simulink model "MCLV_V2_33EP256MC506_LongHurstMotor_sensored_V2"  (R2019a)
settings: Solver=FixedStepDiscrete  StartTime=0.0  StopTime=inf  FixedStep=.01  RelTol=1e-3  EnableMultiTasking=on
undefined symbols (not defined in the file or in its folder): A4, A8, B15, B9, C5, C6, D5, D8, F1, Max, MaxPer, ms, P20, P24, P41, P47, P53, P54, P97, Pin, PWMmax, Resol, us
libraries: MCHP_Blockset x20, simulink x4
(part 1 of 2)
settings Model: SimulationMode=external  ExtModeBatchMode=on  ExtModeTrigDuration=1  Creator=M91449  LastModifiedBy=Lubin Kerhuel
settings DataIOCC: LimitDataPoints=on  ReturnWorkspaceOutputs=off
settings OptimizationCC: DefaultParameterBehavior=Inlined  InlineInvariantSignals=on  LifeSpan=1
settings DebuggingCC: SFUnexpectedBacktrackingDiag=warning  SFNoUnconditionalDefaultTransitionDiag=warning  SFExecutionAtInitializationDiag=none  ArithmeticOperatorsInVariantConditions=warning
settings HardwareCC: ProdBitPerInt=16  ProdBitPerPointer=16  ProdBitPerSizeT=16  ProdBitPerPtrDiffT=16  ProdLargestAtomicInteger=Integer  ProdLargestAtomicFloat=None  ProdWordSize=16  ProdHWDeviceType=Generic->Custom
settings ModelReferenceCC: ModelReferenceNumInstancesAllowed=Single  PropagateSignalLabelsOutOfModel=off
settings SFSimCC: SimUseLocalCustomCode=off  MATLABDynamicMemAlloc=off
settings RTWCC: SystemTargetFile=MCHP_dsPIC_stf.tlc  TemplateMakefile=MCHP_dsPIC.tmf  Description=Microchip Embedded Target PIC24 dsPIC30 dsPIC33 (real-time)  GenerateReport=on  RTWUseLocalCustomCode=off  IncludeHyperlinkInReport=on  LaunchReport=on  GenerateTraceInfo=on  GenerateTraceReport=on  GenerateTraceReportSl=on  GenerateTraceReportSf=on  GenerateTraceReportEml=on  GenerateWebview=on  GenerateCodeMetricsReport=on  GenerateCodeReplacementReport=on
settings CodeAppCC: IgnoreCustomStorageClasses=off  MaxIdLength=255  StateflowObjectComments=on
settings STFCustomTargetCC: TargetLibSuffix=_lib.a  CodeReplacementLibrary=Microchip Code Replacement Library for dsPIC  IncludeMdlTerminateFcn=off  CombineOutputUpdateFcns=on  ERTCustomFileBanners=on  SupportContinuousTime=off  RemoveResetFunc=on  MATLABClassNameForMDSCustomization=Simulink.SoftwareTarget.ERTCustomization  GRTInterface=off  SystemTargetFile=MCHP_dsPIC_stf.tlc
settings ERTTargetCC: TargetLibSuffix=_lib.a  CodeReplacementLibrary=Microchip Code Replacement Library for dsPIC  MultiwordLength=2048  ParMdlRefBuildCompliant=off  CompOptLevelCompliant=off  ConcurrentExecutionCompliant=off  IncludeMdlTerminateFcn=off  SupportNonInlinedSFcns=on  ModelStepFunctionPrototypeControlCompliant=off  CPPClassGenCompliant=off  UseToolchainInfoCompliant=off  ExtMode=on  ExtModeStaticAlloc=on  ExtModeStaticAllocSize=512  ExtModeMexFile=ext_serial_win32_comm_no_acks  ExtModeMexArgs=1 4 115200  InlinedParameterPlacement=NonHierarchical  ERTSrcFileBannerTemplate=MCHP_dsPIC_code_template.cgt  ERTHdrFileBannerTemplate=MCHP_dsPIC_code_template.cgt  ERTDataSrcFileTemplate=MCHP_dsPIC_code_template.cgt  ERTDataHdrFileTemplate=MCHP_dsPIC_code_template.cgt  ERTCustomFileTemplate=MCHP_main.tlc  ConvertIfToSwitch=off  SuppressUnreachableDefaultCases=off
settings ConfigComp: CovMetricSettings=dw  CovHtmlReporting=on  CovSaveCumulativeToWorkspaceVar=on  CovSaveSingleToWorkspaceVar=on  CovExternalEMLEnable=off

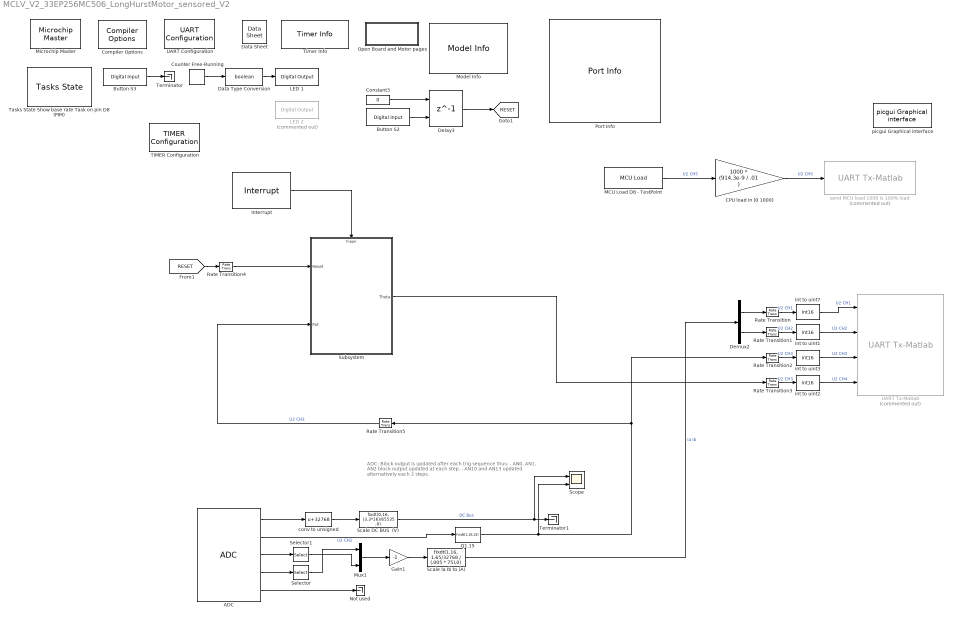
== system MCLV_V2_33EP256MC506_LongHurstMotor_sensored_V2 ==
  note: ADC:
      | Block output is updated after each trig sequence thus:
      | - AN0, AN1, AN2 block output updated at each step.
      | - AN10 and AN13 updated alternatively each 2 steps.
  ADC : MCHP_Blockset/Analog IO/ADC  Priority=5  ADC_REF=1  Mode=10 bits (allows exact simultaneous sampling)  FORM="sddd dddd dddd 0000  ==> Signed fractional"  ADC_R="< 5    kOhm"  nSAMPLECHANNELS=CH0 : CH1 : CH2 : CH3  nSAMPLECHANNELS_12bits=CH0 only  SIMULTANEOUS=Simultaneously on all Channels  ADxCSS=[10 13]  MUXA_CH0N=off  MUXA_CH123=Dynamic Options  MUXA_CH123_TXT=AN0 : AN1 : AN2  MUXB_CH0=AN1  MUXB_CH0N=on  MUXB_CH123=Dynamic Options  MUXB_CH123_TXT=AN0 : AN1 : AN2  SequenceRepeat=1  SequenceTiming=are done as fast as possible ; triggered by user define source  SSRC_SSRCG=Dynamic Options  SSRC_SSRCG_TXT=6  Update_BlockOutput=After all trig and conversion sequence  Trig_TimeStep=not synchronised with ADC [timer based...]  ADC_DMA_CHANNEL=Use Interrupt instead of DMA  SampleTime=0.01  Info=Total Time for Sample & Conversion : 8.9143e-06s including 3.4286e-07s (x 2) sample time.  MCHP_PORT={Analog Input 0}{AN0}15:2:A0;{Analog Input 1}{AN1}15:2:A1;{Analog Input 2}{AN2}15:2:B0;{Analog Input 10}{AN10}15:2:A12;{Analog Input 13}{AN13}15:2:E13;  MCHP_MASTERLINK=MCLV_V2_33EP256MC506_LongHurstMotor_sensored_V2/Microchip Master  ADC_TIMING=[8.9142857142857143663e-06]
      settings: SourceProductName=MPLAB Device Blocks for Simulink
  Button S2 : MCHP_Blockset/Digital IO/Digital Input  PORT=Dynamic Options  PORT_TXT="G   [ 6 : 9 ]"  PIN=7  PACK=off  SIMULTANEOUS=off  ORDERING=None  SampleTime=-1  MCHP_PORT={Digital In}{DIN}2:0:G7;  MCHP_MASTERLINK=MCLV_V2_33EP256MC506_LongHurstMotor_sensored_V2/Microchip Master
      settings: SourceProductName=MPLAB Device Blocks for Simulink
  Button S3 : MCHP_Blockset/Digital IO/Digital Input  PORT=Dynamic Options  PORT_TXT="G   [ 6 : 9 ]"  PIN=6  PACK=off  SIMULTANEOUS=off  ORDERING=None  SampleTime=.1  MCHP_PORT={Digital In}{DIN}2:0:G6;  MCHP_MASTERLINK=MCLV_V2_33EP256MC506_LongHurstMotor_sensored_V2/Microchip Master
      settings: SourceProductName=MPLAB Device Blocks for Simulink
  CPU load in [0 1000] : Gain  Gain=1000 * (914.3e-9 / .01 )  OutDataTypeStr=uint16
  Compiler Options : MCHP_Blockset/System Configuration/Compiler Options  Priority=1  LATEST_CMPLR=on  COMP_LIST=Dynamic Options  COMP_LIST_TXT=xc16 - v1.36  USE_64BIT_DOUBLE=off  MCHP_MULTITHREAD_COMPILATION=on  UseCustom_LinkerScript=off  MCHP_MASTERLINK=MCLV_V2_33EP256MC506_LongHurstMotor_sensored_V2/Microchip Master  OPTIMIZATION_LEVEL=3  OPTIMIZATION_FLTO=on  OPTIMIZATION_REORDER=off  UNROLL_LOOPS=on  PROCEDURAL_ABSTRACTION=off  MPLAB_LINKLIB=default  MPLAB_LINKLIB1=default  MCODE=is less than 32768 (faster)  MCONST=in data memory  MDATA=Use only memory below address 8192 (faster)  MSCALAR=Use only memory below address 8192 (faster)  MLARGEARRAY=off  MAGGREGATE=off  HEAP_SIZE=0  OMF=elf  DEBUG_INFO=off  ProduceHexOutput=on  AssemblyListing=off  NO_EDS_WARN=on  PRINT_STATISTICS=off
      settings: SourceProductName=MPLAB Device Blocks for Simulink
  Constant3 : Constant  Value=0  OutDataTypeStr=uint16  SampleTime=-1
  Counter Free-Running : simulink/Sources/Counter Free-Running  NumBits=1  tsamp=.1
  Data Sheet : MCHP_Blockset/System Info/Data Sheet  DOC_Type=datasheet  DOC_MCHP_Id=33EP256MC506_datasheet  DOC_FilePath=C:\Users\M91449\AppData\Local\Temp\70000657H.pdf  DOC_FileLastCheckTime="[2016              1             28             13             25         44.133]"  cpy_MCHP_Id=33EP256MC506  MCHP_MASTERLINK=MCLV_V2_33EP256MC506_LongHurstMotor_sensored_V2/Microchip Master
      settings: AttributesFormatString=%<cpy_MCHP_Id>  SourceProductName=MPLAB Device Blocks for Simulink
  Data Type Conversion : DataTypeConversion  OutDataTypeStr=boolean
  Delay3 : Delay  DelayLength=1  InitialCondition=1  ExternalReset=Falling  SampleTime=.1
      settings: InputPortMap=u0,r5
  Demux2 : Demux  Outputs=2
  Gain1 : Gain  Gain=-1  SaturateOnIntegerOverflow=on  OutDataTypeStr=Inherit: Same as input
  Interrupt : MCHP_Blockset/System Functions/Interrupt  Interruption=Dynamic Options  Interruption_TXT=TimerA  InterruptionLongDesc=TimerA  IntPriority=5  IntPriority_Info=5  StartupExecute=on  Status=OK  MCHP_MASTERLINK=MCLV_V2_33EP256MC506_LongHurstMotor_sensored_V2/Microchip Master  FPUNoSave=on  Triggered_Sub_TimeSource=is derived from model base rate  TrigsPeriod=0  TIMER_Resolution=Dynamic Options  TIMER_Resolution_TXT="Resol: 0.01429(us)  -  MaxPer: 0.936(ms)"  Info=0  SS_ASYNCHRONOUS_INTERRUPT=0  SS_TIMESOURCE=1  SS_AsyncTimerRes=-1  SS_AsyncTaskPriority=5  SS_ARCH=16
      settings: SourceProductName=MPLAB Device Blocks for Simulink
  LED 1 : MCHP_Blockset/Digital IO/Digital Output  PORT=Dynamic Options  PORT_TXT="D   [ 5  6  8 ]"  PIN=6  PACK=off  SIMULTANEOUS=off  READPREVIOUS=off  ORDERING=None  SampleTime=-1  MCHP_MASTERLINK=MCLV_V2_33EP256MC506_LongHurstMotor_sensored_V2/Microchip Master
      settings: SourceProductName=MPLAB Device Blocks for Simulink
  LED 2 : MCHP_Blockset/Digital IO/Digital Output  Commented=on  PORT=Dynamic Options  PORT_TXT="D   [ 5  6  8 ]"  PIN=5  PACK=off  SIMULTANEOUS=off  READPREVIOUS=off  ORDERING=None  SampleTime=-1  MCHP_MASTERLINK=MCLV_V2_33EP256MC506_LongHurstMotor_sensored_V2/Microchip Master
      settings: SourceProductName=MPLAB Device Blocks for Simulink
  MCU Load D8 - TestPoint : MCHP_Blockset/Profiling/MCU Load  MCULoadPin=Dynamic Options  MCULoadPin_TXT=D5 / Pin[53]  MCULoadMeasure=on  TIMER_Resolution=Dynamic Options  TIMER_Resolution_TXT="Resol: 0.9143(us)  -  Max: 59.9(ms)"  MCHP_PORT={MCU Load Pin}{MCU_Load}0:1:D5;  MCHP_TIMER_REQUEST={MCU_Load}{MCU_Load}21:5:0:0:[]:4194304;  MCHP_TIMER_RESULT=[3 65535 ]  MCHP_MASTERLINK=MCLV_V2_33EP256MC506_LongHurstMotor_sensored_V2/Microchip Master  MCHP_COMPILED_INFO="CompiledSampleTime= [0.010000000000000000208   0 ];CompiledInportDataTypes=[ ];CompiledInportDataWidth=[];"  Info="Timer 3:  Resol: 914.2857143(ns)  -  Max: 59.9186(ms)"  SampleTime=.01
      settings: SourceProductName=MPLAB Device Blocks for Simulink
  Microchip Master : MCHP_Blockset/System Configuration/Microchip Master  Priority=1  PICREF=33EP256MC506  TIMESTEP_REF="Timer  ( 0.01s + [-0.0045714%] ==> 0.0099995s )"  BUSYFLAG=Dynamic Options  BUSYFLAG_TXT=D8 / Pin[42]  PWRTEN=Not used  BOREN=Disable  BODENV=2.7V  BORV=Not used  FPWRT=128ms  DSBOREN=Enable ZPBOR during Deep Sleep Mode  DSLPBOR=Not used  MCLRE=Enabled  SMCLR=MCLR pin generates a normal system Reset  PMDL1WAY=Allow only one reconfiguration  RSTPRI=Device will obtain reset instruction from Primary flash  TEMP=Not used  SOSCSRC=Not used  SOSCSEL=Not used  IOL1WAY=Allow only one reconfiguration  ALTVREF=Not used  DISUVREG=Not used  DSSWEN=Not used  LPCFG=Not used  RTCBAT=Not used  VBTBOR=Not used  WUTSEL=Not used  POWERSAVE=off  FNOSC=Primary Oscillator (XT; HS; EC)  FPR=ECIO w/ PLL 16x  FOSFPR=HS3 w/PLL 16x  FOS=Primary Oscillator  FRANGE=High Range  OSCILLATOR_SELECT=Crystal / Ceramic resonator  OSCILLATOR_SELECT_spd=Crystal / Ceramic resonator  QUARTZ=8e6  QUARTZ_spd=8e6  POSCGAIN=2x gain setting  POSCBOOST=Boost the kick start of the oscillator  SOSCGAIN=2x gain setting  SOSCBOOST=Boost the kick start of the oscillator  ACTIV_PLL=on  ACTIV_PLL_spd=on  MIPS_DESIRED=70e6  MIPS_DESIRED_spd=70e6  FPLLMUL=Not used  FPLLIDIV=8x Divider  POSCFREQ=Not used  POSCMD=XT Crystal Oscillator Mode  POSCMOD=Primary Oscillator Disabled  MIPS=70 * 1e6  ACLKCON=Optimized for PWM resolution & ADC conversion speed  FPLLODIV=32x Divider  PLLKEN=Clock switch to PLL source will wait until the PLL lock signal is valid.  FCKSM=Both Clock switching and Fail-safe Clock Monitor are enabled  FCKSMEN=Sw Disabled; Mon Disabled  IESO=Start up with FRC; then switch  DSWDTPS=1:2^36  FWDTEN=Disable  FWDTWINSZ=Window size is 25%  FWPSA=1:512  FWPSA0=1:128  FWPSB=1:16  WDT=Disable  WDTPOST=1:32768  WDTPRE=1:128  WDTPS=1:32768  WINDIS=Watchdog Timer in Non-Window mode  WWDTEN=Non-Window mode  DSWDTEN=Enable DSWDT during Deep Sleep Mode  DSWDTOSC=Select LPRC as DSWDT Reference clock  FPBDIV=Not used  FSOSCEN=Enable SOSC  LPRCSEL=Not used  OSCIOFCN=Not used  OSCIOFNC=general purpose digital I/O pin  LVRCFG=Not used  PLL_96MHZ=Not used  PLL96MHZ=Not used  PLLDIV=Not used  WDTCLK=Not used  WDTCMX=Not used  WDTWIN=WDT Window is 25% of WDT period  XTCFG=24-32 MHz crystals  XTBST=Boost the kick-start  APL=Aux Flash Code protect is disabled  APLK=Aux Flash Write Protection or Code Protection is Enabled  AWRP=Auxiliary program memory is not write-protected  BSS=No Boot program Flash segment  BWP=Not used  BWRP=Boot Segment may be written  CP=Protection Disabled  EBS=No Boot EEPROM  ESS=No Segment Data EEPROM  GCP=General Segment Code protect is Disabled  GSS=General Segment Code protect is Disabled  GSS0=Not used  GSSK=General Segment Write Protection or Code Protection is Enabled  GWRP=General Segment may be written  PWP=Not used  RBS=No Boot RAM  RSS=No Secure RAM  SSS=No Secure Segment  SWRP=Secure segment may be written  WPCFG=Not used  WPDIS=Not used  WPEND=Not used  WPFP=Not used  ICESEL=Communicate on PGEC1/PGED1  ICS=Communicate on PGEC2 and PGED2  JTAGEN=Disable  COE=Not used  RES=Not used  DEBUG=Debugger is disabled  BACKBUG=Not used  BKBUG=Not used  ALTI2C=I2C mapped to SDA1/SCL1 pins  ALTI2C1=I2C1 mapped to SDA1/SCL1 pins  ALTI2C2=I2C2 mapped to SDA2/SCL2 pins  ALTI2C3=I2C3 mapped to SDA3/SCL3 pins  ALTQIO=QEA1; QEB1; INDX1 are selected as inputs to QEI1  ALTSS1=SS1A is selected as the I/O pin for SPI1  CMPPOL0=Hysteresis is applied to falling edge  CMPPOL1=Hysteresis is applied to falling edge  FCANIO=Not used  FETHIO=Default Ethernet I/O  FMIIEN=MII Enabled  FSRSSEL=Not used  FUSBIDIO=Controlled by the USB Module  FVBUSONIO=Not used  HPOL=PWM module high side output pins have active-high output polarity  HYST0=45 mV Hysteresis  HYST1=45 mV Hysteresis  I2C1SEL=Not used  LPOL=PWM module low side output pins have active-high output polarity  PWMPIN=PWM module pins controlled by PORT register at device Reset  RTCOSC=Not used  UPLLEN=USB PLL Disabled  UPLLIDIV=Not used  ATMOD8=Not used  ALTPMP=Not used  I2C2SEL=Not used  ALTADREF=Not used  ALTCVREF=Not used  PWMLOCK=PWM registers may be written without key sequence  INT_PRIORITY_DMA=0  MCHP_TIMER_REQUEST={Time Step}{TS}0:2:3:1:[]:700000;  MCHP_TIMER_RESULT=[1 10936.499999999987267 ]  MCHP_PORT={Busy Flag}{Busy}0:1:D8;  MCHP_PLLRegisters="[5    243  16385     -1     -1]"  MCHPVAR=MCHP.fcy.MIPS=70000000;MCHP.fcy.SYSCLK=70000000;MCHP.fcy.ADC=70000000;MCHP.fcy.Comparator=70000000;MCHP.fcy.I2C=70000000;MCHP.fcy.SPI=70000000;MCHP.fcy.UART=70000000;MCHP.fcy.Timers=70000000;MCHP.fcy.OC=70000000;MCHP.fcy.IC=70000000;MCHP.fcy.Ports=70000000;MCHP.fcy.QEI=70000000;MCHP.PowerSave=0;MCHP.TimeStepFactor=MCHP_Fun.Hex2num('3FEFFFA0215469B2');MCHP.TimeStep_Timer=1;MCHP.NTIMERS=5;MCHP.id.name='33EP256MC506';MCHP.id.N=reshape([33 256 506],1,3);MCHP.id.L=reshape({ 'EP','MC',''},1,3);MCHP.id.Arch=3;MCHP.periph.PPS.reg_RPINRx=reshape([-1 1 1 -1 -1 -1 1 -1 -1 -1 -1 -1 -1 -1 1 1 1 1 -1 -1 -1 -1 -1 -1 1 1 -1 -1 1 1 1 1 -1 -1 -1 -1 1 -1 1 -1 -1 -1 -1 -1 1 1 1 -1 -1 -1 -1 -1 1 -1 -1 -1 -1 -1 -1 -1 -1 -1 -1 -1 -1 -1 -1 -1 -1 -1 -1 -1 -1 -1 -1 1 -1 1 1 1],1,80);MCHP.PPS.dsPIC.RP=reshape([-1 -1 -1 -1 -1 -1 -1 -1 -1 -1 -1 -1 -1 -1 -1 -1 -1 -1 -1 -1 4 -1 -1 -1 -1 -1 -1 -1 -1 -1 -1 -1 -1 -1 -1 19 20 21 22 23 24 25 26 27 -1 -1 -1 -1 -1 -1 -1 -1 -1 -1 38 39 40 41 -1 -1 -1 -1 -1 -1 -1 -1 -1 -1 -1 -1 -1 -1 -1 -1 -1 -1 -1 -1 -1 -1 -1 -1 -1 -1 -1 -1 -1 -1 -1 -1 -1 -1 -1 -1 -1 -1 -1 81 -1 -1 -1 -1 -1 -1 -1 -1 -1 -1 -1 -1 -1 -1 -1 -1 -1 -1 -1 -1 102 -1 104],1,121);MCHP.PPS.dsPIC.RPI=reshape([-1 -1 -1 -1 -1 -1 -1 -1 -1 -1 -1 -1 -1 -1 -1 -1 -1 -1 -1 -1 -1 -1 -1 -1 8 9 -1 11 12 -1 -1 -1 16 17 18 -1 -1 -1 -1 -1 -1 -1 -1 -1 28 29 30 31 -1 -1 -1 35 36 37 -1 -1 -1 -1 42 -1 -1 -1 -1 -1 -1 -1 -1 -1 -1 -1 -1 -1 -1 -1 -1 -1 -1 -1 -1 -1 -1 -1 -1 -1 -1 -1 -1 -1 -1 -1 -1 -1 -1 -1 78 79 80 -1 -1 -1 -1 -1 -1 -1 -1 -1 -1 -1 -1 -1 -1 -1 -1 -1 -1 -1 -1 -1 -1 103 -1 105],1,122);MCHP.PPS.dsPIC.RPINR_list=reshape({ '1','INT1','INT2','INT3','INT4','T1CK','T2CK','T3CK','T4CK','T5CK','T6CK','T7CK','T8CK','T9CK','IC1','IC2','IC3','IC4','IC5','IC6','IC7','IC8','OCFA','OCFB','FLT1','FLT2','FLT3','FLT4','QEIA1','QEIB1','QEINDX1','QEIHOM1','QEIA2','QEIB2','QEINDX2','QEIHOM2','U1RX','U1CTS','U2RX','U2CTS','SDI1','SCK1_in','SS1_in','44','SDI2','SCK2_in','SS2_in','48','CSDIR','CSCK','COFS','52','C1RX','C2RX','U3RX','U3CTS','U4RX','U4CTS','SDI3','SCK3_in','SS3_in','62','SDI4','SCK4_in','SS4_in','66','IC9','IC10','IC11','IC12','IC13','IC14','IC15','IC16','OCFC','SYNCI1','SYNCI2','DTCMP1','DTCMP2','DTCMP3','DTCMP4','DTCMP5','DTCMP6','DTCMP7','FLT5','FLT6','FLT7','FLT8','89','SENT1','SENT2','92'},1,92);MCHP.PPS.dsPIC.RPOR_list=reshape({ '1','U1TX','U1RTS','U2TX','U2RTS','SDO1','SCK1_out','SS1_out','SDO2','SCK2_out','SS2_out','CSDO','CSCK','COFS','C1TX','C2TX','OC1','OC2','OC3','OC4','OC5','OC6','OC7','OC8','C1OUT','C2OUT','C3OUT','U3TX','U3RTS','U4TX','U4RTS','SDO3','SCK3_out','SS3_out','SDO4','SCK4_out','SS4_out','OC9','OC10','OC11','OC12','OC13','OC14','OC15','OC16','SYNCO1','SYNCO2','QEI1CCMP','QEI2CCMP','REFCLK','C4OUT','C5OUT','52','53','54','55','56','SENT1','SENT2'},1,59);MCHP.PPS.map_RPnR_RPORx=reshape([20 35 36 37 38 39 40 41 42 43 54 55 56 57 -1 97 -1 118 120],1,19);MCHP.Rx=reshape([13 15 21 -1 -1 58 -1 -1 -1 -1 -1 14 16 22 -1 -1 59 -1 -1 -1 -1 -1 -1 17 23 -1 -1 -1 -1 -1 -1 -1 -1 -1 18 35 -1 -1 -1 -1 -1 -1 -1 -1 33 32 36 -1 -1 -1 -1 -1 -1 -1 -1 -1 43 37 53 -1 -1 -1 -1 -1 -1 -1 -1 44 50 54 -1 -1 4 -1 -1 -1 -1 1 46 51 -1 -1 -1 5 -1 -1 -1 -1 31 48 52 42 -1 -1 6 -1 -1 -1 -1 34 49 55 -1 -1 -1 8 -1 -1 -1 -1 64 60 45 -1 -1 -1 -1 -1 -1 -1 -1 12 61 24 -1 -1 -1 -1 -1 -1 -1 -1 11 62 39 -1 27 -1 -1 -1 -1 -1 -1 -1 63 47 -1 28 -1 -1 -1 -1 -1 -1 -1 2 -1 -1 29 -1 -1 -1 -1 -1 -1 -1 3 40 -1 30 -1 -1 -1 -1 -1 -1],11,16);MCHP.ADC.ANtype=reshape([3 0],1,2);MCHP.ADC.ADCONx=reshape([47103 59391 40959 263 0 0],1,6);MCHP.ADC.ADCHS_0=reshape([40863 1799],1,2);MCHP.ADC.Flags=reshape([1 0],1,2);MCHP.ADC.Buffer=reshape([16 -1],1,2);MCHP.ADC.port=reshape([0 1 16 17 18 19 32 33 34 11 12 43 76 77 78 79 -1 -1 -1 -1 -1 -1 -1 -1 -1 -1 -1 -1 -1 -1 -1 -1 -1 -1 -1 -1 -1 -1 -1 -1 -1 -1 -1 -1 -1 -1 -1 -1 -1 -1 -1 -1 -1 -1 -1 -1 -1],1,57);MCHP.ADC.port_ALT=reshape([-1 -1 -1 -1],1,4);MCHP.ADC.port_VrefP=17;MCHP.ADC.port_VrefM=16;MCHP.ADC.port_AVdd=-1;MCHP.ADC.port_AVss=-1;MCHP.ADC.ADCDATA=reshape([0 0 0 0 0 0 0 0 0 0 0 0 0 0 0 0 0 0 0 0 0 0 0 0 0 0 0 0 0 0 0 0 0 0 0 0 0 0 0 0 0 0 0 0 0 0 0 0 0 0 0 0 0 0 0 0 0],1,57);MCHP.ADC.HS_SAR.TRGSRC=reshape([0 0 0 0 0 0 0 0 0 0 0 0 0 0 0 0 0 0 0 0 0 0 0 0 0 0],1,26);MCHP.ADC.HS_SAR.nFilters=0;MCHP.ADC.HS_SAR.nDedicatedCore=0;MCHP.ADC.HS_SAR.CALIBRATION=0;MCHP.ADC.HS_SAR.ADCON1L=-1;MCHP.memory.RAM=32768;MCHP.memory.RAM_XBegin=4096;MCHP.memory.RAM_YBegin=20480;MCHP.memory.RAM_dma=reshape([-1 -1],1,2);MCHP.memory.FLASH_ECC=0;MCHP.DMA.Num=4;MCHP.DMA.CNTmax=16383;MCHP.QEI.QEICONx=reshape([49023 -1 -1 -1 -1 -1],1,6);MCHP.QEI.QEItype=1;MCHP.QEI.Port_QEI_INDX=reshape([-1 -1],1,2);MCHP.QEI.Port_QEI_QEA=reshape([-1 -1],1,2);MCHP.QEI.Port_QEI_QEB=reshape([-1 -1],1,2);MCHP.QEI.Port_QEI_UPDN=reshape([-1 -1],1,2);MCHP.INT.Port=reshape([23 32767 32767 -1 -1],1,5);MCHP.PWM_HS.Flags=reshape([3 1 0],1,3);MCHP.PWM.port_FLT=reshape([-1 -1 -1 34 43 -1 -1 -1 -1 -1 -1 -1 -1 -1 -1 -1 -1 -1 -1 -1 -1 -1 -1 -1 -1 -1 -1 -1 -1 -1 -1 -1 20],1,33);MCHP.PWM.PWMRef=-1;MCHP.PWM.Flag=0;MCHP.PWM.Port_PWM_l=reshape([31 -1 29 -1 27 -1 -1 -1 -1 -1 -1 -1 -1 -1 -1 -1 -1 -1 -1 -1 -1 -1 -1 -1],2,12);MCHP.PWM.Port_PWM_h=reshape([30 -1 28 -1 26 -1 -1 -1 -1 -1 -1 -1 -1 -1 -1 -1 -1 -1 -1 -1 -1 -1 -1 -1],2,12);MCHP.PWM_HS_FEP.nEVTOUT=-1;MCHP.IC.Port=reshape([32767 32767 32767 32767 0 0 0 0 0 0 0 0 0 0 0 0],1,16);MCHP.IC.type=1;MCHP.OC.Port=reshape([32767 32767 32767 32767 0 0 0 0 0 0 0 0 0 0 0 0],1,16);MCHP.OC.type=1;MCHP.CN.Port=reshape([-1 -1 -1 -1 -1 -1 -1 -1 -1 -1 -1 -1 -1 -1 -1 -1 -1 -1 -1 -1 -1 -1 -1 -1 -1 -1 -1 -1 -1 -1 -1 -1 -1 -1 -1 -1 -1 -1 -1 -1 -1 -1 -1 -1 -1 -1 -1 -1 -1 -1 -1 -1 -1 -1 -1 -1 -1 -1 -1 -1 -1 -1 -1 -1 -1 -1 -1 -1 -1 -1 -1 -1 -1 -1 -1 -1 -1 -1 -1 -1 -1 -1 -1 -1 -1],1,85);MCHP.CN.PullUp=reshape([8083 65535 49151 352 61440 3 960 0 0 0 0],1,11);MCHP.CN.type=1;MCHP.CN.Flag_PullDown=1;MCHP.SPI.Refs=reshape([1 2 0 0 0 0],1,6);MCHP.SPI.SPIxCON1=8191;MCHP.SPI.SPIxCON2=57347;MCHP.SPI.Port_SDI=reshape([9 -1 -1 -1 -1 -1],1,6);MCHP.SPI.Port_SDO=reshape([4 -1 -1 -1 -1 -1],1,6);MCHP.SPI.Port_SCK=reshape([35 -1 -1 -1 -1 -1],1,6);MCHP.SPI.Port_SS=reshape([16 -1 -1 -1 -1 -1],1,6);MCHP.I2C.Refs=reshape([1 2 0 0 0],1,5);MCHP.I2C.I2CxCON=49151;MCHP.I2C.NewRegName=1;MCHP.I2C.Port_SDA=reshape([36 8 -1 -1 -1],1,5);MCHP.I2C.Port_SCL=reshape([37 20 -1 -1 -1],1,5);MCHP.I2C.Port_ASDA=reshape([25 21 -1 -1 -1],1,5);MCHP.I2C.Port_ASCL=reshape([24 22 -1 -1 -1],1,5);MCHP.I2C.Fuse_Port_SCL_SDA=reshape([3 1 4 1 -1 -1 -1 -1 -1 -1],2,5);MCHP.I2C.Fuse_Port_ASCL_ASDA=reshape([3 2 4 2 -1 -1 -1 -1 -1 -1],2,5);MCHP.SCCP.nSCCP=0;MCHP.SCCP.MCCP=reshape([0 0 0 0 0 0 0 0 0],1,9);MCHP.PGA.Port_PGA1P=reshape([-1 -1 -1 -1],1,4);MCHP.PGA.Port_PGA1N=reshape([-1 -1 -1 -1],1,4);MCHP.PGA.Port_PGA2P=reshape([-1 -1 -1 -1],1,4);MCHP.PGA.Port_PGA2N=reshape([-1 -1 -1 -1],1,4);MCHP.PGA.Num=2;MCHP.HS_AnalogComparator.Port_CMP1=reshape([-1 -1 -1 -1],1,4);MCHP.HS_AnalogComparator.Port_CMP2=reshape([-1 -1 -1 -1],1,4);MCHP.HS_AnalogComparator.Port_CMP3=reshape([-1 -1 -1 -1],1,4);MCHP.HS_AnalogComparator.Port_CMP4=reshape([-1 -1 -1 -1],1,4);MCHP.HS_AnalogComparator.PORT_EXTREFx=reshape([-1 -1],1,2);MCHP.HS_AnalogComparator.Port_DACOUTx=reshape([-1 -1],1,2);MCHP.HS_AnalogComparator.Num=2;MCHP.Comp.Port_CVrefin=-1;MCHP.Comp.Port_CVref=-1;MCHP.Comp.Port_CVref1O=24;MCHP.Comp.Port_CVref2O=4;MCHP.Comp.Port_CxOUT=reshape([32767 32767 32767 32767 -1],1,5);MCHP.Comp.Port_OAxOUT=reshape([17 0 32 -1 -1],1,5);MCHP.Comp.Port_CxINP=reshape([18 1 34 32 -1],1,5);MCHP.Comp.Port_CxINM=reshape([19 43 -1 -1 16 76 -1 -1 33 77 -1 -1 33 -1 -1 -1 -1 -1 -1 -1],4,5);MCHP.Comp.Port_OAxINP=reshape([-1 -1 -1 -1 -1],1,5);MCHP.Comp.Port_OAxINM=reshape([-1 -1 -1 -1 -1],1,5);MCHP.Comp.nComp=reshape([4 0 0],1,3);MCHP.Comp.OpAmp=7;MCHP.Comp.CVRCON=reshape([17663 0],1,2);MCHP.CDAC.Port_DACx=reshape([-1 -1 -1],1,3);MCHP.CDAC.nCDAC=0;MCHP.UART.port_Rx=reshape([32767 32767 -1 -1 -1 -1],1,6);MCHP.UART.port_Tx=reshape([32767 32767 -1 -1 -1 -1],1,6);MCHP.UART.port_ARx=reshape([-1 -1],1,2);MCHP.UART.port_ATx=reshape([-1 -1],1,2);MCHP.UART.port_RTS=reshape([34 76 -1 -1 -1 -1],1,6);MCHP.UART.port_CTS=reshape([43 77 -1 -1 -1 -1],1,6);MCHP.UART.reg_UxMODE=reshape([48127 48127 -1 -1 -1 -1],1,6);MCHP.UART.reg_UxSTA=reshape([61439 61439 -1 -1 -1 -1],1,6);MCHP.modsrc.DOS_02551_cpu_16bit_v7=0;MCHP.modsrc.DOS_01520_wdt_dmt_upb_v1_16bit=0;MCHP.modsrc.DOS_02359a_sent_j2716_upb_v1=0;MCHP.modsrc.DOS_02672_math_progcrc_upb_v1_16bit=0;MCHP.modsrc.DOS_01577_cla_clc_upb_v1=0;MCHP.modsrc.DOS_02915_ecc_v2=0;MCHP.modsrc.DOS_02673_tmr_classa_upb_v1_16bit=0;MCHP.modsrc.DOS_01494_qei_32b_upb_v1_16bit=0;MCHP.modsrc.DOS_02552_msi_upb_v1_Master=0;MCHP.modsrc.DOS_01441_i2c_upb_v1_16bit_TLAH=0;MCHP.modsrc.DOS_03076_uart_protocol_upb_v1_16bit=0;MCHP.modsrc.DOS_01482=0;MCHP.modsrc.DOS_01483_pwm_16bit=0;MCHP.modsrc.DOS_03247_CAN_FD_UPB_V2_16_bit=0;MCHP.modsrc.DOS_02497_WACV=0;MCHP.modsrc.DOS_02316_nvm_ctrl_v1_16bit=0;MCHP.modsrc.DOS_02653_afe_current_bias_ctrl_upb_v1_16bit=0;MCHP.modsrc.DOS_01459_ptg_pc_upb_v1_16bit=0;MCHP.modsrc.DOS_01512_ccp_mccp_upb_v1_16bit=0;MCHP.modsrc.DOS_02519_dma_sfr_16bit_v2=0;MCHP.modsrc.DOS_02508c11=0;MCHP.modsrc.DOS_02475_dac_pdm_nbit_upb_v1_16bit=0;MCHP.modsrc.DOS_02467_gpio_upb_v1_16bit=0;MCHP.modsrc.DOS_00805_rst_integration_v4=0;MCHP.modsrc.DOS_02659_clk_sib_v12=0;MCHP.modsrc.DOS_02674_wdt_upb_v1_16bit=0;MCHP.modsrc.DOS_01407=0;MCHP.modsrc.DOS_02552_msi_upb_v1_Slave=0;MCHP.modsrc.DOS_02593_amp_pga_ctrl_pb_v2_16bit=0;MCHP.modsrc.DOS_01461_afe_ctmu_con_upb_v1_16bit=0;MCHP.modsrc.DOS_02497_WACA=0;MCHP.modsrc.DOS_02478_uart_irda_upb_v1_16bit=0;MCHP.modsrc.DOS_00929=1;MCHP.modsrc.DOS_01198=1;MCHP.modsrc.DOS_03029_WACH=0;MCHP.modsrc.DOS_02472_ppi_pmp16_upb_v1_16bit=0;MCHP.modsrc.DOS_02949_WACG=0;MCHP.modsrc.DOS_03349_amp_pad_opamp_ctrl_upb_v1=0;MCHP.modsrc.DOS_02237_osc_dco_ctrl_upb_v1_16bit=0;MCHP.modsrc.DOS_03662_WACU=0;MCHP.modsrc.DOS_03994_WAC07_Module=0;MCHP.modsrc.DOS_00794=1;MCHP.modsrc.DOS_00931=1;MCHP.modsrc.DOS_00932=1;MCHP.modsrc.DOS_00942=1;MCHP.modsrc.DOS_00938=1;MCHP.modsrc.DOS_00996=1;MCHP.modsrc.DOS_00997=1;MCHP.modsrc.DOS_00998=1;MCHP.modsrc.DOS_00209=0;MCHP.modsrc.DOS_01555_adc=0;MCHP.modsrc.DOS_01293=1;MCHP.modsrc.DOS_00828=0;MCHP.modsrc.DOS_01116=1;MCHP.modsrc.DOS_01017_RPORx=1;MCHP.modsrc.DOS_01017_RPINRx=1;MCHP.modsrc.DOS_01555_nvm_tsmc18_v2_16bit=0;MCHP.modsrc.DOS_00804=1;MCHP.modsrc.DOS_00826=1;MCHP.modsrc.DOS_01555_TLAK_PMDx=0;MCHP.modsrc.DOS_01555_TLAK_INT_=0;MCHP.modsrc.DOS_00933=1;MCHP.modsrc.DOS_01555=0;MCHP.modsrc.DOS_01555_ptg=0;MCHP.modsrc.DOS_00958=1;MCHP.modsrc.DOS_01117_PORTx=1;MCHP.modsrc.DOS_00999=0;MCHP.modsrc.DOS_01041=1;MCHP.modsrc.DOS_00892=1;MCHP.modsrc.DOS_01287_TLAC_PMDx=1;MCHP.modsrc.DOS_01287_TLAC_INT_=1;MCHP.modsrc.DOS_01424=1;MCHP.modsrc.DOS_01332=1;MCHP.modsrc.DOS_01468_PMBA_current_source=0;MCHP.modsrc.DOS_02291_PGA=0;MCHP.modsrc.DOS_01467_Comparator=0;MCHP.modsrc.DOS_01498_TLAY=0;MCHP.modsrc.DOS_00993_PLL_120MHz=0;MCHP.modsrc.DOS_01332_ptg_pc_v1=0;MCHP.modsrc.DOS_00958_pwm_TLAY=0;MCHP.modsrc.TLAY_IOPorts=0;MCHP.modsrc.DOS_00929q=0;MCHP.modsrc.DOS_02415_spi_v5=0;MCHP.modsrc.DOS_RPINRx_16bit_2=0;MCHP.modsrc.DOS_01497_TLAH_PMDx=0;MCHP.modsrc.DOS_02550_TLAL_INT=0;MCHP.modsrc.DOS_00958_pwm_TLAH=0;MCHP.modsrc.DOS_01287_TLAH_INT_=0;MCHP.modsrc.DOS_01113=0;MCHP.modsrc.DOS_01017_PMDx=0;MCHP.modsrc.DOS_00927=0;MCHP.modsrc.DOS_01080=0;MCHP.modsrc.DOS_00794_cpu_16bit_v3=0;MCHP.modsrc.DOS_02192_TLCD_PMDx=0;MCHP.modsrc.DOS_02192_TLCD_INT_=0;MCHP.modsrc.DOS_02192_cmp=0;MCHP.modsrc.DOS_00958_pwm_TLCD=0;MCHP.modsrc.DOS_02192_PORTx_TLCD=0;MCHP.modsrc.DOS_00936=0;MCHP.modsrc.DOS_00995=0;MCHP.modsrc.DOS_00546=0;MCHP.modsrc.DOS_00474=0;MCHP.modsrc.DOS_02481_WACJ_MC_Config=0;MCHP.modsrc.DOS_02569_pfm_cache_ocp_v1=0;MCHP.modsrc.DOS_02819_pfm_ctrl_32bit_upb_v2=0;MCHP.modsrc.DOS_02674_wdt_upb_v1_32bit=0;MCHP.modsrc.DOS_01520_wdt_dmt_upb_v1=0;MCHP.modsrc.DOS_02869_icd_jtag_bvci_upb_v2=0;MCHP.modsrc.DOS_02823_WACJ_clk_cru_upb_v2=0;MCHP.modsrc.DOS_01423_RPINRx=0;MCHP.modsrc.DOS_02481_RPORx=0;MCHP.modsrc.DOS_02511_pwr_sib_upb_v1_32bit=0;MCHP.modsrc.DOS_02481_WACJ_MC_int_evic_v3=0;MCHP.modsrc.DOS_01500_dma_bvci_v2=0;MCHP.modsrc.DOS_02141_tmr_classa_pb_v2=0;MCHP.modsrc.DOS_02815_tmr_classb_upb_v1=0;MCHP.modsrc.DOS_00740_icap_pb_v1=0;MCHP.modsrc.DOS_00749_ocmp_pb_v1=0;MCHP.modsrc.DOS_01441_i2c_upb_v1_32bit=0;MCHP.modsrc.DOS_01329_spi_pb_v2=0;MCHP.modsrc.DOS_02478_uart_irda_upb_v1_32bit=0;MCHP.modsrc.DOS_02514_dfm_strl_sst_upb_v1=0;MCHP.modsrc.DOS_01477_pwm_mc_upb_v1=0;MCHP.modsrc.DOS_01459_ptg_pc_upb_v1_SIC=0;MCHP.modsrc.DOS_01494_qei_32b_upb_v1=0;MCHP.modsrc.DOS_01427_cmp_control_upb_v1_32bit=0;MCHP.modsrc.DOS_01445_dac_nbit__control_upb_v1_32bit=0;MCHP.modsrc.DOS_01461_afe_ctmu_con_upb_v1=0;MCHP.modsrc.DOS_02472_ppi_pmp16_upb_v1=0;MCHP.modsrc.DOS_02467_gpio_ports_upb_v1=0;MCHP.modsrc.DOS_01152_can_bvci_v1=0;MCHP.modsrc.DOS_02508_adc_sar_ctrl_upb_v1_PIC32MK=0;MCHP.modsrc.DOS_02813a_usb_otgcore_pb_v3=0;MCHP.modsrc.DOS_01261_tmr_rtcc_pb_v2=0;MCHP.modsrc.DOS_01475_lpwr_deep_sleep_ctrl_v2=0;MCHP.modsrc.DOS_EIP_00136_ssx_v1=0;MCHP.modsrc.DOS_02481_WACK_MC_Config=0;MCHP.modsrc.DOS_03088_pfm_cache_ocp_v2_WACK=0;MCHP.modsrc.DOS_02823_WACN_clk_cru_upb_v2=0;MCHP.modsrc.DOS_02907_WACK_MC_int_evic_v3=0;MCHP.modsrc.DOS_03554_cmp_control_upb_v2_32bit=0;MCHP.modsrc.DOS_03247_can_fd_upb_v2_pic32mk=0;MCHP.modsrc.DOS_02787_WACD_Config=0;MCHP.modsrc.DOS_00800_dac_4bit_ctrl_pb_v1=0;MCHP.modsrc.DOS_01539_icd_jtag_pb_v2=0;MCHP.modsrc.DOS_02823_clk_cru_upb_v2=0;MCHP.modsrc.DOS_01423_RPORx=0;MCHP.modsrc.DOS_02907_WACD_int_evic_v3=0;MCHP.modsrc.DOS_00734_uart_irda_pb_v1=0;MCHP.modsrc.DOS_00687_tmr_classa_pb_v1=0;MCHP.modsrc.DOS_00745_tmr_classb_pb_v1=0;MCHP.modsrc.DOS_02508_adc_sar_ctrl_upb_v1=0;MCHP.modsrc.DOS_00866_cmp_control_pb_v2=0;MCHP.modsrc.DOS_01114_eth_bvci_v1=0;MCHP.modsrc.DOS_02831_usb_clk_rst_v2=0;MCHP.modsrc.DOS_01643_pfm_cache_ahb_v2=0;MCHP.modsrc.DOS_EIP_00206r5_sqi_v2=0;MCHP.modsrc.DOS_EIP_00124_usb_hs_otgcore_v1=0;MCHP.modsrc.DOS_EIP_00218_math_rng_ahbs_v2=0;MCHP.modsrc.DOS_EIP_00109_ebi_v1=0;MCHP.modsrc.DOS_EIP_00158_crypto_v1=0;MCHP.PortBase=16;MCHP.PortPrefixe='P';MCHP.clock.PBxDIV=-1;  MCHP_CRC=6863099  BTMODE=Not used  RES1=Not used  PLLSS=Not used  RES2=Not used  ALTCMPI=Not used  BOREN1=Not used  ALTRB6=Not used  RETCFG=Not used  DFMCY=Not used  BSS2=No Boot Segment  BSEN=No Boot Segment  CWRP=Configuration Segment may be written  CSS=No Protection (other than CWRP)  AIVTDIS=Disable Alternate Vector Table  BSLIM=Not used  WDTEN=Disable  BTSWP=BOOTSWP instruction is disabled  DBCC=No Cross Connection between DAC outputs  CTXT1=Not Assigned  CTXT2=Not Assigned  SEQNUM=Not used  nSEQNUM=Not used  BOREN0=Enabled  DMTIVT=Not used  DMTCNT=2^31 (2147483648)  DMTEN=Dead Man Timer is Disabled and can be enabled by software  ON=Not used  USERID=Not used  RESERVED1=Not used  PGL1WAY=Allow only one reconfiguration  FPLLRNG=34-68 MHz Input  FPLLICLK=FRC is input to the System PLL  FPLLMULT=PLL Multiply by 128  UPLLFSEL=USB PLL input is 24 MHz  DMTINTV=Window/Interval value is 127/128 counter value  WDTSPGM=WDT stops during Flash programming  FDMTEN=Deadman Timer is disabled  TRCEN=Trace features in the CPU are enabled  BOOTISA=Boot code and Exception code is MIPS32  FECCCON=ECC and Dynamic ECC are disabled (ECCCON bits are writable)  EXTDDRSIZE=Not used  FSLEEP=Flash is powered down when the device is in Sleep mode  DBGPER=Allow CPU access to all permission regions  EJTAGBEN=Normal EJTAG functionality  TSEQ=Not used  CSEQ=Not used
      settings: SourceProductName=MPLAB Device Blocks for Simulink
  Model Info : simulink/Model-Wide Utilities/Model Info  Frame=on  DisplayStringWithTags=|  HorizontalTextAlignment=Left  LeftAlignmentValue=0.02
      | Long hust motor with:
      | M1 - Black
      | M2 - Red
      | M3 - White
      | 
      | Encoder on HA - HB 
      | HA: Blue wire
      | HB: White wire
  Mux1 : Mux  Inputs=2
  Not used : Terminator
  Open Board and Motor pages : Subsystem
      settings: OpenFcn=|
      | web('www.microchip.com/DevelopmentTools/ProductDetails.aspx?PartNO=DM330021-2','-browser');
      | pause(1);
      | web('http://www.microchipdirect.com/productsearch.aspx?keywords=AC300020','-browser');
      | pause(1);
      | web('www.microchipdirect.com/ProductSearch.aspx?keywords=AC300022','-browser');
      mask Display: disp('Open tools\nWebpage');
  Port Info : MCHP_Blockset/System Info/Port Info  MCHP_MASTERLINK=MCLV_V2_33EP256MC506_LongHurstMotor_sensored_V2/Microchip Master
      settings: SourceProductName=MPLAB Device Blocks for Simulink
  Q1.15 : DataTypeConversion  OutDataTypeStr=fixdt(1,16,15)  ConvertRealWorld=Stored Integer (SI)
  Rate Transition : RateTransition
  Rate Transition1 : RateTransition
  Rate Transition2 : RateTransition
  Rate Transition3 : RateTransition  Deterministic=off
  Rate Transition4 : RateTransition  Deterministic=off
  Rate Transition5 : RateTransition  Deterministic=off
  Scale DC BUS  (V) : DataTypeConversion  OutDataTypeStr=fixdt(0,16, (3.3*16)/65535 ,0)  ConvertRealWorld=Stored Integer (SI)
  Scale Ia Ib to (A) : DataTypeConversion  OutDataTypeStr=fixdt(1,16, 1.65/32768 / (.005 * 75),0)  ConvertRealWorld=Stored Integer (SI)
  Scope : Scope  NumInputPorts=2
  Selector : Selector  InputPortWidth=2  IndexOptions=Index vector (dialog)  Indices=2  OutputSizes=1
  Selector1 : Selector  InputPortWidth=2  IndexOptions=Index vector (dialog)  Indices=2  OutputSizes=1
  Subsystem : Subsystem
  TIMER Configuration : MCHP_Blockset/Timers/TIMER Configuration  TIMER_Name=TimerA  TIMER_CustomName=pouet_p  TIMER_Ressource=Dynamic Options  TIMER_Ressource_TXT=No constraints [Prefered]  TIMER_Ressource_Custom=[1]  DoNotSetupChk=off  TIMER_PeriodChk=off  TIMER_Period=50e-6  TIMER_Resolution=Dynamic Options  TIMER_Resolution_TXT="Resol: 3.657(us)  -  MaxPer: 240(ms)"  TIMER_Interrupt=off  TIMER_Use=Read only  TIMER_ShareChk=on  MCHP_TIMER_REQUEST="{TimerA}{TmrCfg}20:2:3:0:[1  2  3  4  5]:3500;"  MCHP_TIMER_RESULT=[2 3498.9999999999990905 ]  MCHP_USER_INTERRUPTS={T2}{TimerA}{TimerA}{VectorName(T2Interrupt) Priority(-1) };  MCHP_MASTERLINK=MCLV_V2_33EP256MC506_LongHurstMotor_sensored_V2/Microchip Master  Info="Timer 2:  Resol: 14.28571429(ns)  -  Per: 50(us)  -  Max value: 936.214(us)"
      settings: SourceProductName=MPLAB Device Blocks for Simulink
  Tasks State Show base rate Task on pin D8 (PIM) : MCHP_Blockset/Profiling/Tasks State  TasksPin=D8  MCHP_PORT={Task D1 Running}{Task D1}15:1:D8;  MCHP_MASTERLINK=MCLV_V2_33EP256MC506_LongHurstMotor_sensored_V2/Microchip Master
      settings: SourceProductName=MPLAB Device Blocks for Simulink
  Terminator : Terminator
  Terminator1 : Terminator
  Timer Info : MCHP_Blockset/System Info/Timer Info  MCHP_MASTERLINK=MCLV_V2_33EP256MC506_LongHurstMotor_sensored_V2/Microchip Master
      settings: SourceProductName=MPLAB Device Blocks for Simulink
  UART Configuration : MCHP_Blockset/BUS UART/UART Configuration  UART_REF=2  BAUD_Choice=Dynamic Options  BAUD_Choice_TXT="115200         [-0.06%]"  BAUD_Choice_IR=Dynamic Options  BAUD_Choice_IR_TXT=[]  BAUD_Custom=115200  INT_PRIORITY=0  ALT_IO=on  PIN_RX=Dynamic Options  PIN_RX_TXT=C5 / P53 / Pin[37]  PIN_TX=Dynamic Options  PIN_TX_TXT=F1 / P97 / Pin[59]  MCHP_PORT="{UART2  Rx}{U2RX}3:0:P53;{UART2  Tx}{U2TX}3:1:P97;"  MCHP_MASTERLINK=MCLV_V2_33EP256MC506_LongHurstMotor_sensored_V2/Microchip Master  MCHP_COM_ExtPil=on  TX_IMPLEMENTATION=Circular Buffer  TX_IMPLEMENTATION_default=Circular Buffer  TX_INT_PRIORITY=5  TX_INT_WHEN=is empty & last char is sent  TX_INT_WHEN_default=is empty & last char is sent  TX_CIRCULAR_SIZE=256  TX_DMA_CHANNEL="0   (Lowest Priority)"  TX_DMA_SIZE=60  TX_TASK_PROTECTION=Delay tasks (default)  TX_INTERRUPT_PROTECTION=Do not send on conflict (default)  TX_INTERRUPT_PROTECTION_default=Do not send on conflict (default)  RX_IMPLEMENTATION=Circular Buffer  RX_IMPLEMENTATION_default=Circular Buffer  RX_INT_PRIORITY=5  RX_INT_WHEN=is 3/4 fulll (contains 3 data characters)  RX_CIRCULAR_SIZE=256  RX_DMA_CHANNEL=0  RX_DMA_SIZE=0  DuplexMode=Full duplex (default)  PIN_RX_Inv=off  PIN_TX_Inv=off  PIN_RXTX_Inv=off  ParityBit=No parity (default)  StopBit=1 stop bit (default)  IRDA=off  FlowControl=None  PIN_CTS=Dynamic Options  PIN_CTS_TXT=A4 / P20 / Pin[33]  PIN_RTS=Dynamic Options  PIN_RTS_TXT=A4 / P20 / Pin[33]  InitSequence_chkbox=off  BAUD_Choice_InitSeq=Dynamic Options  BAUD_Choice_InitSeq_TXT="110         [-0.00%]"  BAUD_Choice_IR_InitSeq=Dynamic Options  BAUD_Choice_IR_InitSeq_TXT=0  BAUD_Custom_InitSeq=0  InitSequence='Hello World'
      settings: SourceProductName=MPLAB Device Blocks for Simulink
  UART Tx-Matlab : MCHP_Blockset/BUS UART/UART Tx-Matlab  Commented=on  UART_REF=2  CHANNELS=[1 2 3 4 ]  AllOrNothing=on  SampleTime=.001  MCHP_MASTERLINK=MCLV_V2_33EP256MC506_LongHurstMotor_sensored_V2/Microchip Master  MCHP_COMPILED_INFO="CompiledSampleTime= [0.0010000000000000000208   0 ];CompiledInportDataTypes=[  4   4   4   4 ];CompiledInportDataWidth=[1  1  1  1];"
      settings: SourceProductName=MPLAB Device Blocks for Simulink
  conv to unsigned : Bias  Bias=32768
  int to uint{1..3,7} (4 alike) : DataTypeConversion  OutDataTypeStr=int16  ConvertRealWorld=Stored Integer (SI)
  picgui Graphical interface : MCHP_Blockset/BUS UART/picgui Graphical interface  Nothing=0
      settings: SourceProductName=MPLAB Device Blocks for Simulink
  send MCU load 1000 is 100% load : MCHP_Blockset/BUS UART/UART Tx-Matlab  Commented=on  UART_REF=2  CHANNELS=5  AllOrNothing=on  SampleTime=-1  MCHP_MASTERLINK=MCLV_V2_33EP256MC506_LongHurstMotor_sensored_V2/Microchip Master  MCHP_COMPILED_INFO="CompiledSampleTime= [0.0050000000000000001041   0 ];CompiledInportDataTypes=[  5 ];CompiledInportDataWidth=[1];"
      settings: SourceProductName=MPLAB Device Blocks for Simulink
  tag scope: RESET=global
  wires:
  Counter Free-Running/1 -> Data Type Conversion/1
  Data Type Conversion/1 -> LED 1/1
  Rate Transition/1 -> int to uint7/1  "U2 CH1"
  Rate Transition1/1 -> int to uint1/1  "U2 CH2"
  Constant3/1 -> Delay3/1
  Rate Transition2/1 -> int to uint3/1  "U2 CH3"
  Delay3/1 -> [RESET]
  int to uint3/1 -> UART Tx-Matlab/3  "U2 CH3"
  [RESET] -> Rate Transition4/1
  int to uint1/1 -> UART Tx-Matlab/2  "U2 CH2"
  int to uint7/1 -> UART Tx-Matlab/1  "U2 CH1"
  CPU load in [0 1000]/1 -> send MCU load 1000 is 100% load/1  "U2 CH5"
  Button S3/1 -> Terminator/1
  Demux2/1 -> Rate Transition/1
  Demux2/2 -> Rate Transition1/1
  Button S2/1 -> Delay3/2
  int to uint2/1 -> UART Tx-Matlab/4  "U2 CH4"
  Rate Transition3/1 -> int to uint2/1  "U2 CH3"
  Rate Transition4/1 -> Subsystem/1(Reset)
  Subsystem/1(Theta) -> Rate Transition3/1
  Interrupt/1 -> Subsystem/Trigger
  MCU Load D8 - TestPoint/1 -> CPU load in [0 1000]/1  "U2 CH5"
  Selector1/1 -> Mux1/2
  ADC/4 -> Selector/1
  ADC/3 -> Selector1/1
  Gain1/1 -> Scale Ia Ib to (A)/1
  ADC/5 -> Not used/1
  ADC/1 -> conv to unsigned/1
  conv to unsigned/1 -> Scale DC BUS  (V)/1
  ADC/2 -> Q1.15/1  "U2 CH2"
  Mux1/1 -> Gain1/1
  Selector/1 -> Mux1/1
  Q1.15/1 -> Scope/2, Rate Transition2/1, Rate Transition5/1
  Scale Ia Ib to (A)/1 -> Demux2/1  "Ia Ib"
  Rate Transition5/1 -> Subsystem/2(Pot)  "U2 CH3"
  Scale DC BUS  (V)/1 -> Scope/1, Terminator1/1  "DC Bus"

== system MCLV_V2_33EP256MC506_LongHurstMotor_sensored_V2/Open Board and Motor pages ==

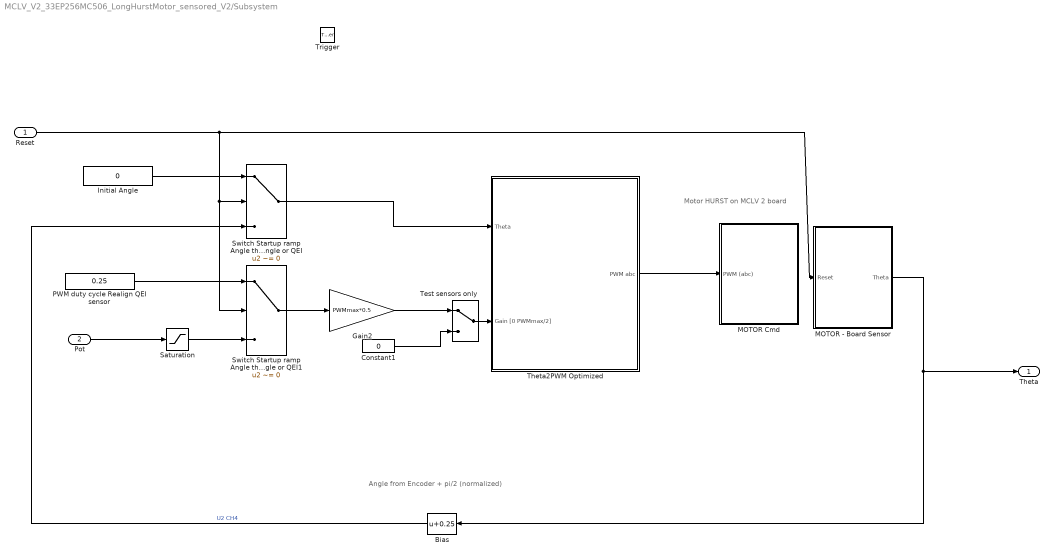
== system MCLV_V2_33EP256MC506_LongHurstMotor_sensored_V2/Subsystem ==
  note: Motor HURST on MCLV 2 board
  note: Angle from Encoder + pi/2 (normalized)
  Reset : Inport
  Pot : Inport  Port=2
  Trigger : TriggerPort  TriggerType=function-call  VariantControl=Variant  PortDimensions=1
  Bias : Bias  Bias=0.25
  Constant1 : Constant  Value=0  OutDataTypeStr=Inherit: Inherit via back propagation  SampleTime=-1
  Gain2 : Gain  Gain=PWMmax*0.5  OutMin=-PWMmax*0.5  OutMax=PWMmax*0.5  OutDataTypeStr=fixdt(1,16)
  "Initial Angle " : Constant  Value=0  OutDataTypeStr=Inherit: Inherit via back propagation
  MOTOR Cmd : Subsystem
  MOTOR - Board Sensor : Subsystem
  PWM duty cycle Realign QEI sensor : Constant  Value=0.25  OutDataTypeStr=Inherit: Inherit via back propagation
  Saturation : Saturate  UpperLimit=1  LowerLimit=-1
  Switch Startup ramp Angle then Estimated Angle or QEI : Switch  Criteria=u2 ~= 0  Threshold=250
  Switch Startup ramp Angle then Estimated Angle or QEI1 : Switch  Criteria=u2 ~= 0  Threshold=250
  Test sensors only : ManualSwitch
  Theta2PWM Optimized : Subsystem  VariantControl=Optimized
  Theta : Outport
  wires:
  Saturation/1 -> Switch Startup ramp Angle then Estimated Angle or QEI1/3
  Theta2PWM Optimized/1(PWM abc) -> MOTOR Cmd/1(PWM (abc))
  MOTOR - Board Sensor/1(Theta) -> Theta/1, Bias/1
  Test sensors only/1 -> Theta2PWM Optimized/2(Gain [0 PWMmax/2])
  Constant1/1 -> Test sensors only/2
  Switch Startup ramp Angle then Estimated Angle or QEI1/1 -> Gain2/1
  Switch Startup ramp Angle then Estimated Angle or QEI/1 -> Theta2PWM Optimized/1(Theta)
  Reset/1 -> MOTOR - Board Sensor/1(Reset), Switch Startup ramp Angle then Estimated Angle or QEI1/2, Switch Startup ramp Angle then Estimated Angle or QEI/2
  "Initial Angle "/1 -> Switch Startup ramp Angle then Estimated Angle or QEI/1
  Bias/1 -> Switch Startup ramp Angle then Estimated Angle or QEI/3  "U2 CH4"
  PWM duty cycle Realign QEI sensor/1 -> Switch Startup ramp Angle then Estimated Angle or QEI1/1
  Gain2/1 -> Test sensors only/1
  Pot/1 -> Saturation/1

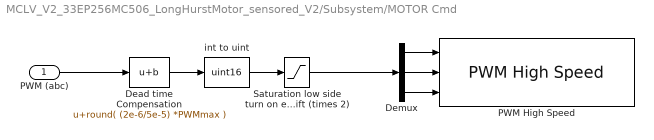
== system MCLV_V2_33EP256MC506_LongHurstMotor_sensored_V2/Subsystem/MOTOR Cmd ==
  PWM (abc) : Inport
  Dead time Compensation : Bias  Bias=round( (2e-6/5e-5) *PWMmax )
  Demux : Demux  Outputs=3
  PWM High Speed : MCHP_Blockset/PWM IO/PWM High Speed  pop1=[1]  chk1="[1  1  1  0  0]"  chkHL1="[1  1  1  1  1  1  1  1 ; 1  1  1  1  1  1  1  1]"  maxP1={ '5e-05','5e-05','5e-05','0.001','0.001','0.001','0.001','0.001';'0.001','0.001','1e-06','0.001','0.001','0.001','0.001','0.001'}  InitP2={ '5e-05','5e-05','5e-05','0.001','0.001','0.001','0.001','0.001';'0.001','0.001','0.001','0.001','0.001','0.001','0.001','0.001'}  chkP2="[0  0  0  1  1  1  1  1 ; 1  0  0  1  1  1  1  1]"  InitDC={ '4','4','4','50','50','50','50','50';'0.001','0.001','0.001','50','50','50','50','50'}  chkDC="[1  1  1  1  1  1  1  1 ; 0  0  0  1  1  1  1  1]"  InitPh={ '0','0','0','0.001','0.001','0.001','0.001','0.001';'0','0','0','0.001','0.001','0.001','0.001','0.001'}  chkPh="[0  0  0  1  1  1  1  1 ; 0  0  0  1  1  1  1  1]"  edSEvTrigx={ '0','-1','-1','-1','-1','-1','-1','-1'}  chkSEvTrigx="[0  0  0  1  1  1  1  1]"  popFlt="[2  2  2  1  1  1  1  1]"  popFltPin="[20  20  20   4   4   4   4   4]"  popFltPinRp="[1  1  1  1  1  1  1]"  popFltActivH="[2  2  2  1  1  1  1  1]"  popFltForceH="[2  2  2  2  2  2  2  2]"  popFltForceL="[1  1  1  1  1  1  1  1]"  chkFltBlkOut="[0  0  0  0  0  0  0  0]"  popIndepFaultMode="[1  1  1  1  1  1  1  1]"  popCurEnabled="[1  1  1  1  1  1  1  1]"  popCurPin="[4  31   4   4   4   4   4   4]"  popCurActiveH="[1  1  1  1  1  1  1  1]"  popCurForceH="[2  1  2  1  1  1  1  1]"  popCurForceL="[2  1  2  1  1  1  1  1]"  ChkCurBlkOut="[1  0  0  0  0  0  0  0]"  ChkCurBlkOutTime="[1  0  1  0  0  0  0  0]"  popBLANKSEL="[1  1  1  1  1  1  1  1]"  popBPHHBPHL="[1  1  1  1  1  1  1  1]"  popBPLHBPLL="[1  1  1  1  1  1  1  1]"  popFLTLEBEN_CLLEBEN="[1  1  1  1  1  1  1  1]"  popPHR_PHF="[2  1  1  1  1  1  1  1]"  popPLR_PLF="[3  1  1  1  1  1  1  1]"  edLEB={ '100e-9','50e-9','150e-9','50e-9','50e-9','50e-9','50e-9','50e-9'}  popDT="[1  1  1  3  3  3  3  3]"  edDTRx={ '0','0','0','1e-05','1e-05','1e-05','1e-05','1e-05'}  edAltDTRx={ '2e-06','2e-06','2e-06','1e-05','1e-05','1e-05','1e-05','1e-05'}  S_INPUT="[5  5  5]"  S_INPUT_Size="[1  1  1]"  S_OUTPUT=[]  S_OUTPUT_Size=[]  S_DWORK_Type=[]  S_DWORK_Size=[]  ADC_VARTRIG={PWM Primary Special Event Trigger;6}  evalin_ws=PWMmax = 3499;PWM1max = 3499;PWM2max = 3499;PWM3max = 3499;  SampleTime=-1  ORDERING=None  MCHP_PORT={PWM1 Fault}{FLT32}4:0:B4;{PWM2 Fault}{FLT32}4:0:B4;{PWM3 Fault}{FLT32}4:0:B4;{PWM1H}{PWM1H}4:4:B14;{PWM1L}{PWM1L}4:4:B15;{PWM2H}{PWM2H}4:4:B12;{PWM2L}{PWM2L}4:4:B13;{PWM3H}{PWM3H}4:4:B10;{PWM3L}{PWM3L}4:4:B11;  MCHP_MASTERLINK=MCLV_V2_33EP256MC506_LongHurstMotor_sensored_V2/Microchip Master  MCHP_VERSION=v3.38  Parameter50=0
      settings: SourceProductName=MPLAB Device Blocks for Simulink
  Saturation low side turn on errate workaround + errata for Phase shift (times 2) : Saturate  UpperLimit=PWMmax  LowerLimit=round( (2e-6/5e-5) *PWMmax )* 2
  int to uint : DataTypeConversion  OutDataTypeStr=uint16  ConvertRealWorld=Stored Integer (SI)
  wires:
  Demux/1 -> PWM High Speed/1
  Demux/3 -> PWM High Speed/3
  Demux/2 -> PWM High Speed/2
  int to uint/1 -> Saturation low side turn on errate workaround + errata for Phase shift (times 2)/1
  Saturation low side turn on errate workaround + errata for Phase shift (times 2)/1 -> Demux/1
  Dead time Compensation/1 -> int to uint/1
  PWM (abc)/1 -> Dead time Compensation/1

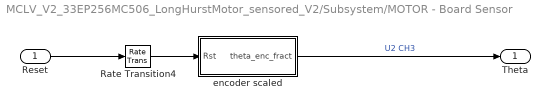
== system MCLV_V2_33EP256MC506_LongHurstMotor_sensored_V2/Subsystem/MOTOR - Board Sensor ==
  Reset : Inport
  Rate Transition4 : RateTransition  InitialCondition=1
  encoder scaled : Subsystem
  Theta : Outport
  wires:
  encoder scaled/1(theta_enc_fract) -> Theta/1  "U2 CH3"
  Rate Transition4/1 -> encoder scaled/1(Rst)
  Reset/1 -> Rate Transition4/1

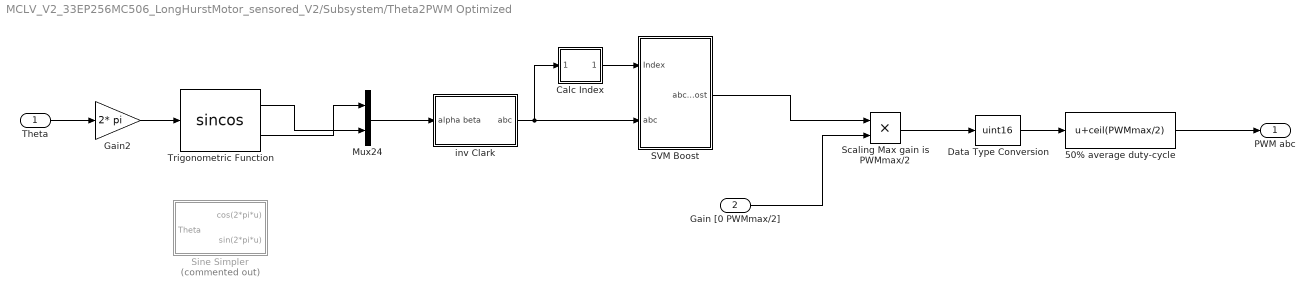
== system MCLV_V2_33EP256MC506_LongHurstMotor_sensored_V2/Subsystem/Theta2PWM Optimized ==
  Theta : Inport  OutDataTypeStr=fixdt(0,16,16)
  Gain [0 PWMmax/2] : Inport  Port=2  OutMin=[-PWMmax/2]  OutMax=[PWMmax/2]
  50% average duty-cycle : Bias  Bias=ceil(PWMmax/2)
  Calc Index : Subsystem
  Data Type Conversion : DataTypeConversion  OutDataTypeStr=uint16  ConvertRealWorld=Stored Integer (SI)
  Gain2 : Gain  Gain=2* pi  OutDataTypeStr=fixdt(0,16,13)  RndMeth=Convergent
  Mux24 : Mux  Inputs=2
  SVM Boost : Subsystem
  Scaling Max gain is PWMmax/2 : Product  Inputs=**  OutDataTypeStr=int16
  Sine Simpler : Subsystem  Commented=on
  Trigonometric Function : Trigonometry  Operator=sincos  ApproximationMethod=CORDIC  NumberOfIterations=15
  inv Clark : Subsystem
  PWM abc : Outport
  wires:
  Mux24/1 -> inv Clark/1(alpha beta)
  Scaling Max gain is PWMmax/2/1 -> Data Type Conversion/1
  Gain [0 PWMmax/2]/1 -> Scaling Max gain is PWMmax/2/2
  Calc Index/1(Idx) -> SVM Boost/1(Index)
  inv Clark/1(abc) -> Calc Index/1(In1), SVM Boost/2(abc)
  Theta/1 -> Gain2/1
  SVM Boost/1(abc boost) -> Scaling Max gain is PWMmax/2/1
  50% average duty-cycle/1 -> PWM abc/1
  Data Type Conversion/1 -> 50% average duty-cycle/1
  Trigonometric Function/2 -> Mux24/1
  Trigonometric Function/1 -> Mux24/2
  Gain2/1 -> Trigonometric Function/1

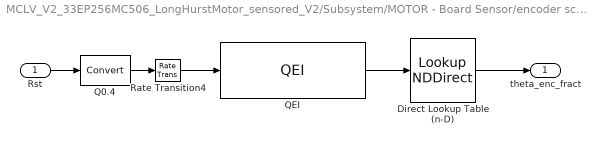
== system MCLV_V2_33EP256MC506_LongHurstMotor_sensored_V2/Subsystem/MOTOR - Board Sensor/encoder scaled ==
  Rst : Inport
  Direct Lookup Table (n-D) : LookupNDDirect  NumberOfTableDimensions=1  Table=[0:199]*inv(200)  TableDataTypeStr=fixdt(0,16,16)
      settings: LockScale=on
  Q0.4 : DataTypeConversion
  QEI : MCHP_Blockset/QEI/QEI  QEI_REF=1  QEI_MODE=Quadrature Encoder  QEI_x2mode=off  QEI_PulseCountDir=Down  PIN_QEA=Dynamic Options  PIN_QEA_TXT=C6 / P54 / Pin[50]  PIN_QEB=Dynamic Options  PIN_QEB_TXT=A8 / P24 / Pin[31]  SWPAB=on  QEAPOL=off  QEBPOL=off  SampleTime=-1  PIN_CCMP=Dynamic Options  PIN_CCMP_TXT=A4 / P20 / Pin[33]  MCHP_PORT={QEI1 A}{QEIA1}5:0:P54;{QEI1 B}{QEIB1}5:0:P24;  MCHP_MASTERLINK=MCLV_V2_33EP256MC506_LongHurstMotor_sensored_V2/Microchip Master  INDXxCNT_Output=is not an output  POSxCNT_Output=is a 16 bits unsigned block output  RESET_Input=on  PIMOD_mode=position is cyclique between user defined boundaries  PIMOD_modeB=Never reset position  PIMOD_reset=on next INDEX event  PIN_INDEX=Dynamic Options  PIN_INDEX_TXT=B15 / P47 / Pin[3]  IMV=QEA = 1 and QEB = 0  IMV_x2=QEA = 1  PIN_HOME=Dynamic Options  PIN_HOME_TXT=B9 / P41 / Pin[49]  QEIxLEC_GEC=[0 199]  QEIxIC=0  PCIIRQ=off  IDXPOL=off  HOMPOL=on  VELxCNT_Output=is not an output  INTxHLD_Output=is not an output  MaxPeriod=0.1  FILTREN=on  QFDIV_popup=Dynamic Options  QFDIV_popup_TXT=364.58 kHz  FILTER_CutOffFreq=100e3  QEI_IntPri=5
      settings: SourceProductName=MPLAB Device Blocks for Simulink
  Rate Transition4 : RateTransition  InitialCondition=1
  theta_enc_fract : Outport
  wires:
  Rate Transition4/1 -> QEI/1
  Q0.4/1 -> Rate Transition4/1
  Rst/1 -> Q0.4/1
  Direct Lookup Table (n-D)/1 -> theta_enc_fract/1
  QEI/1 -> Direct Lookup Table (n-D)/1

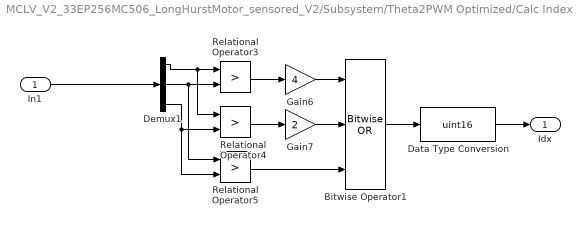
== system MCLV_V2_33EP256MC506_LongHurstMotor_sensored_V2/Subsystem/Theta2PWM Optimized/Calc Index ==
  In1 : Inport
  Bitwise Operator1 : simulink/Logic and Bit Operations/Bitwise Operator  logicop=OR  UseBitMask=off  NumInputPorts=3  BitMask=bin2dec('11011001')  BitMaskRealWorld=Stored Integer
  Data Type Conversion : DataTypeConversion  OutDataTypeStr=uint16  ConvertRealWorld=Stored Integer (SI)
  Demux1 : Demux  Outputs=3
  Gain6 : Gain  Gain=4  OutDataTypeStr=Inherit: Same as input
  Gain7 : Gain  Gain=2  OutDataTypeStr=Inherit: Same as input
  Relational Operator3 : RelationalOperator  Operator=>  OutDataTypeStr=fixdt(1,16)  RndMeth=Nearest
  Relational Operator4 : RelationalOperator  Operator=>  OutDataTypeStr=fixdt(1,16)  RndMeth=Nearest
  Relational Operator5 : RelationalOperator  Operator=>  OutDataTypeStr=fixdt(1,16)  RndMeth=Nearest
  Idx : Outport
  wires:
  Gain7/1 -> Bitwise Operator1/2
  Gain6/1 -> Bitwise Operator1/1
  Relational Operator5/1 -> Bitwise Operator1/3
  Relational Operator3/1 -> Gain6/1
  Demux1/2 -> Relational Operator5/1, Relational Operator3/2
  Demux1/3 -> Relational Operator5/2, Relational Operator4/2
  Relational Operator4/1 -> Gain7/1
  Demux1/1 -> Relational Operator4/1, Relational Operator3/1
  Bitwise Operator1/1 -> Data Type Conversion/1
  In1/1 -> Demux1/1
  Data Type Conversion/1 -> Idx/1

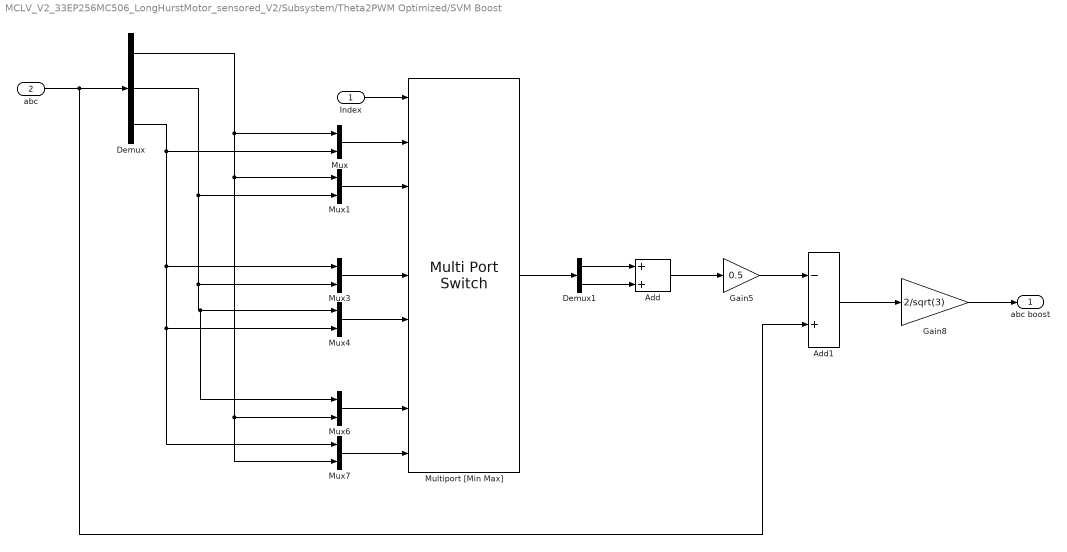
== system MCLV_V2_33EP256MC506_LongHurstMotor_sensored_V2/Subsystem/Theta2PWM Optimized/SVM Boost ==
  Index : Inport
  abc : Inport  Port=2
  Add : Sum  OutDataTypeStr=Inherit: Same as accumulator  RndMeth=Simplest
  Add1 : Sum  Inputs=-+  OutDataTypeStr=Inherit: Same as accumulator  RndMeth=Simplest
  Demux : Demux  Outputs=3
  Demux1 : Demux  Outputs=2
  Gain5 : Gain  Gain=0.5  RndMeth=Simplest  OutDataTypeStr=Inherit: Same as input
  Gain8 : Gain  Gain=2/sqrt(3)  RndMeth=Simplest  OutDataTypeStr=Inherit: Same as input
  Multiport [Min Max] : MultiPortSwitch  DataPortOrder=Zero-based contiguous  Inputs=8  DiagnosticForDefault=None  zeroidx=on
  Mux{,1,3..4,6..7} (6 alike) : Mux  Inputs=2
  abc boost : Outport
  wires:
  Demux1/2 -> Add/2
  Demux1/1 -> Add/1
  Multiport [Min Max]/1 -> Demux1/1
  Demux/2 -> Mux1/2, Mux3/2, Mux4/1, Mux6/1
  Demux/3 -> Mux7/1, Mux4/2, Mux3/1, Mux/2
  Demux/1 -> Mux/1, Mux1/1, Mux6/2, Mux7/2
  Mux7/1 -> Multiport [Min Max]/9
  Mux6/1 -> Multiport [Min Max]/8
  Mux4/1 -> Multiport [Min Max]/6
  Mux3/1 -> Multiport [Min Max]/5
  Mux1/1 -> Multiport [Min Max]/3
  Mux/1 -> Multiport [Min Max]/2
  Index/1 -> Multiport [Min Max]/1
  Gain8/1 -> abc boost/1
  abc/1 -> Demux/1, Add1/2
  Add1/1 -> Gain8/1
  Gain5/1 -> Add1/1
  Add/1 -> Gain5/1
